simulink library "Defined_Functionality"  (R2018a)
settings: Solver=ode45  StartTime=0.0  StopTime=10.0  RelTol=1e-3
undefined symbols (not defined in the file or in its folder): IPTc_dbgsw_pct_RestoreCellSoc, IPTc_dbgval_RestoreCellSoc, IPTc_flter_PosCtrVoltRef1_front, IPTc_Gain_BCSBattVolt, IPTc_Gain_CC2, IPTc_Gain_CMLChagrMaxOptCur, IPTc_Gain_PCBTemp, IPTc_Offset_BCSBattVolt, IPTc_Offset_CC2, IPTc_Offset_CMLChagrMaxOptCur, IPTc_Offset_PCBTemp, IPTc_tm_VehShutBCUCmdDeb, IPTc_v_ChaWake_HysisDnLimit, IPTc_v_ChaWake_HysisUpLimit
settings Model: Creator=Administrator  LastModifiedBy=dhw059
settings DataIOCC: LimitDataPoints=on  SaveFormat=Array  SignalLoggingSaveFormat=ModelDataLogs
settings OptimizationCC: BlockReduction=off  BooleanDataType=off  ExpressionDepthLimit=2147483647  LifeSpan=inf
settings DebuggingCC: SaveWithParameterizedLinksMsg=none  UnderspecifiedInitializationDetection=Classic  MergeDetectMultiDrivingBlocksExec=none  SignalResolutionControl=TryResolveAllWithWarning  FcnCallInpInsideContextMsg=warning  StateNameClashWarn=warning  SFUnexpectedBacktrackingDiag=warning  SFNoUnconditionalDefaultTransitionDiag=warning  SFExecutionAtInitializationDiag=none
settings HardwareCC: ProdBitPerPointer=32  ProdBitPerSizeT=32  ProdBitPerPtrDiffT=32  ProdLargestAtomicFloat=None  ProdIntDivRoundTo=Undefined  ProdEndianess=Unspecified  ProdWordSize=32  ProdHWDeviceType=32-bit Generic  TargetUnknown=on
settings ModelReferenceCC: PropagateSignalLabelsOutOfModel=off
settings CodeAppCC: StateflowObjectComments=on
settings GRTTargetCC: TargetLangStandard=C89/C90 (ANSI)  GeneratePreprocessorConditionals=Disable all  CombineOutputUpdateFcns=off  GRTInterface=on
settings ConfigComp: CovMetricSettings=dw  CovHtmlReporting=on  CovSaveCumulativeToWorkspaceVar=on  CovSaveSingleToWorkspaceVar=on  CovExternalEMLEnable=off

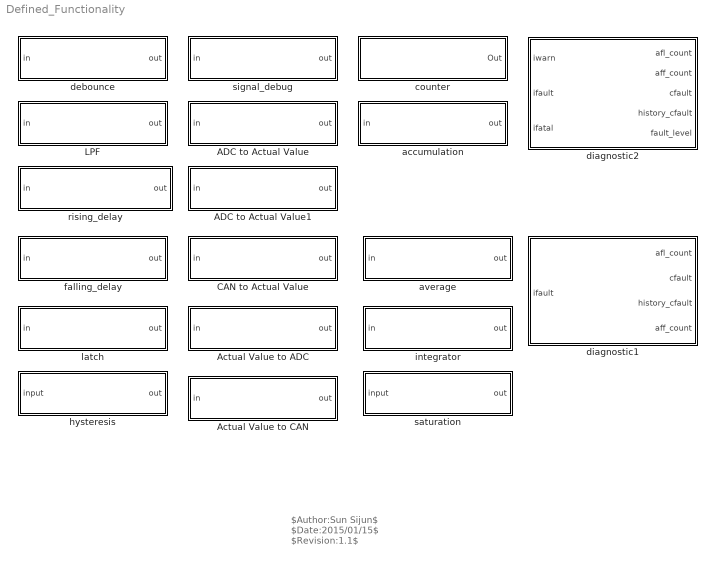
== system Defined_Functionality ==
  note: $Author:Sun Sijun$
      | $Date:2015/01/15$
      | $Revision:1.1$
  ADC to Actual Value : Subsystem  TreatAsAtomicUnit=on  RTWFcnName=ADC_CONVERSION_A_ACT  mask(Value Conversion){gain=IPTc_Gain_CC2, offset=IPTc_Offset_CC2}
      mask help:
      | To convert ADC vaule into actual value.
      | ACT=ADC*GAIN+OFFSET
      settings: AttributesFormatString=[GAIN=%<gain>]\n[OFFSET=%<offset>]  RTWFcnNameOpts=User specified
      mask Display:
      | color('black');
      | disp('CONVERSION_A');
      | port_label('input',1,'ADC')
      | port_label('output',1,'ACT')
  ADC to Actual Value1 : Subsystem  TreatAsAtomicUnit=on  RTWFcnName=ADC_CONVERSION_B_ACT21  mask(Value Conversion){offset=IPTc_Offset_PCBTemp, gain=IPTc_Gain_PCBTemp}
      mask help:
      | To convert ADC vaule into actual value.
      | ACT=(ADC+OFFSET)*GAIN
      settings: AttributesFormatString=[OFFSET=%<offset>]\n[GAIN=%<gain>]  RTWFcnNameOpts=User specified
      mask Display:
      | color('black');
      | disp('CONVERSION_B');
      | port_label('input',1,'ADC')
      | port_label('output',1,'ACT')
  Actual Value to ADC : Subsystem  TreatAsAtomicUnit=on  RTWFcnName=ACT_CONVERSION_ADC  mask(Value Conversion){gain=0, offset=0}
      mask help:
      | To convert actual value into ADC value.
      | ADC=(ACT-OFFSET)/GAIN
      settings: AttributesFormatString=[GAIN=%<gain>]\n[OFFSET=%<offset>]  RTWFcnNameOpts=User specified
      mask Display:
      | color('black');
      | disp('CONVERSION');
      | port_label('input',1,'ACT')
      | port_label('output',1,'ADC')
  Actual Value to CAN : Subsystem  TreatAsAtomicUnit=on  RTWFcnName=ACT_CONVERSION_CAN  mask(Value Conversion){gain=IPTc_Gain_BCSBattVolt, offset=IPTc_Offset_BCSBattVolt}
      mask help: To convert actual value into CAN signal.
      settings: AttributesFormatString=[GAIN=%<gain>]\n[OFFSET=%<offset>]  RTWFcnNameOpts=User specified
      mask Display:
      | color('black');
      | disp('CONVERSION');
      | port_label('input',1,'ACT')
      | port_label('output',1,'CAN')
  CAN to Actual Value : Subsystem  TreatAsAtomicUnit=on  RTWFcnName=CAN_CONVERSION_ACT  mask(Value Conversion){gain=IPTc_Gain_CMLChagrMaxOptCur, offset=IPTc_Offset_CMLChagrMaxOptCur}
      mask help:
      | To convert CAN signal into actual value.
      | ACT=CAN*GAIN+OFFSET.
      settings: AttributesFormatString=[GAIN=%<gain>]\n[OFFSET=%<offset>]  RTWFcnNameOpts=User specified
      mask Display:
      | color('black');
      | disp('CONVERSION');
      | port_label('input',1,'CAN')
      | port_label('output',1,'ACT')
  LPF : Subsystem  TreatAsAtomicUnit=on  RTWFcnName=low_pass_filter2  mask(LPF){filter_gain=IPTc_flter_PosCtrVoltRef1_front}
      mask prompts: filter_gain "LPF_GAIN"
      mask help: Low pass filter.The LPF_GAIN is positive but less than 1.
      settings: AttributesFormatString=[FILTER_GAIN=%<filter_gain>]  RTWFcnNameOpts=User specified
      mask Display:
      | disp('LPF')
      | port_label('input',1,'in')
      | port_label('output',1,'out')
  accumulation : Subsystem  TreatAsAtomicUnit=on  RTWFcnName=accumulation  mask(accumulation){Num_Threshold_Up=200, Num_Threshold_Down=0, Inc=1, Dec=0}
      mask prompts: Num_Threshold_Up "Threshold_Up"; Num_Threshold_Down "Threshold_Down"; Inc "Increment"; Dec "Decrement"
      mask help:
      | The initial output of the block is FALSE.When the input value is TRUE,the counter would increase
      | by Increment value per period,the block will not output TURE until the counter is not less than
      | Threshold.When the input value become FALSE,the counter would decrease by decrement value per
      | period,the block will not output FASLE until the counter is not more than zero.
      settings: AttributesFormatString=[THRESHOLD_UP=%<Num_Threshold_Up>]\n[THRESHOLD_DOWN=%<Num_Threshold_Down>]\n[INCREMENT=%<Inc>]\n[DECREMENT=%<Dec>]  RTWFcnNameOpts=User specified
      mask Display:
      | disp('ACCUMULATION')
      | port_label('input',1,'in')
      | port_label('output',1,'out')
  average : Subsystem  TreatAsAtomicUnit=on  RTWFcnName=average2  mask(average){time=uint16(2000), period=uint16(10)}
      mask prompts: time "Time_ms"; period "Period_ms"
      mask help: To get the average avlue of input signal in the period Time_ms.
      settings: AttributesFormatString=[TIME_ms=%<time>]\n[PERIOD_ms=%<period>]  RTWFcnNameOpts=User specified
      mask Display:
      | port_label('input',1,'in')
      | port_label('output',1,'out')
      | disp('AVERAGE')
  counter : Subsystem  TreatAsAtomicUnit=on  RTWFcnName=counter  mask(counter){initial_value=1, counter_limit=10}
      mask prompts: initial_value "Initial_Counter_Value"
      mask help: The block is a counter.It counts from initial counter value until counter limit,then it will count from initial counter value.
      settings: AttributesFormatString=[INITIAL_VALUE=%<initial_value>]\n[COUNTER_LIMIT=%<counter_limit>]  RTWFcnNameOpts=User specified
      mask Display:
      | disp('COUNTER')
      | port_label('output',1,'out')
  debounce : Subsystem  TreatAsAtomicUnit=on  RTWFcnName=debounce  mask(debounce){debounce_time=IPTc_tm_VehShutBCUCmdDeb}
      mask prompts: debounce_time "debounce_time_ms"
      mask help: Debounce the input digital signal.
      settings: AttributesFormatString=[DEBOUNCE_TIME=%<debounce_time>]  RTWFcnNameOpts=User specified
      mask Display:
      | disp('DEBOUNCE')
      | port_label('input',1,'in')
      | port_label('output',1,'out')
  diagnostic1 : Subsystem  TreatAsAtomicUnit=on  RTWFcnName=diagnostic  mask(Fault_Diagnostic){afl_inc=3, afl_dec=3, afl_threshold=10, aff_threshold=255}
      mask prompts: afl_inc "AFL_INCREMENT"; afl_dec "AFL_DECREMENT"
      mask help:
      | AFL:Accumulated Failure Level.
      | AFF:Accumulated Failure Frequency
      | AFL_INCREMENT:The value of the internal counter gets incremented each cycle if the ifault is active [uint8] [0...255].
      | AFL_DECREMENT:The value of  the internal counter gets decremented each cycle if the ifault is inactive [uint8] [0...255].
      | AFL_THRESHOLD:When the internal counter is more than AFL_THRESHOLD,fault is confirmed.
      | AFF_THRESHOLD:The aff_count must be less than AFF_THRESHOLD.
      settings: AttributesFormatString=[AFL_INCREMENT=%<afl_inc>]\n[AFL_DECREMENT=%<afl_dec>]\n[AFL_THRESHOLD=%<afl_threshold>]\n[AFF_THRESHOLD=%<aff_threshold>]  RTWFcnNameOpts=User specified
      mask Display:
      | disp('DIAGNOSTIC')
      | port_label('input',1,'ifault')
      | port_label('output',1,'afl_count')
      | port_label('output',2,'cfault')
      | port_label('output',3,'history_cfault')
      | port_label('output',4,'aff_count')
  diagnostic2 : Subsystem  TreatAsAtomicUnit=on  RTWFcnName=diagnostic  mask(Fault_Diagnostic){afl_inc=3, afl_dec=3, afl_threshold=10, aff_threshold=255}
      mask prompts: afl_inc "AFL_INCREMENT"; afl_dec "AFL_DECREMENT"
      mask help:
      | AFL:Accumulated Failure Level.
      | AFF:Accumulated Failure Frequency
      | AFL_INCREMENT:The value of the internal counter gets incremented each cycle if the ifault is active [uint8] [0...255].
      | AFL_DECREMENT:The value of  the internal counter gets decremented each cycle if the ifault is inactive [uint8] [0...255].
      | AFL_THRESHOLD:When the internal counter is more than AFL_THRESHOLD,fault is confirmed.
      | AFF_THRESHOLD:The aff_count must be less than AFF_THRESHOLD.
      settings: AttributesFormatString=[AFL_INCREMENT=%<afl_inc>]\n[AFL_DECREMENT=%<afl_dec>]\n[AFL_THRESHOLD=%<afl_threshold>]\n[AFF_THRESHOLD=%<aff_threshold>]  RTWFcnNameOpts=User specified
      mask Display:
      | disp('DIAGNOSTIC')
      | port_label('input',1,'iwarn')
      | port_label('input',2,'ifault')
      | port_label('input',3,'ifatal')
      | port_label('output',1,'afl_count')
      | port_label('output',2,'aff_count')
      | port_label('output',3,'cfault')
      | port_label('output',4,'history_cfault')
      | port_label('output',5,'fault_level')
  falling_delay : Subsystem  TreatAsAtomicUnit=on  RTWFcnName=falling_edge_delay  mask(falling edge delay){delay_time=50}
      mask prompts: delay_time "delay_time_ms"
      mask help: When the input equals TRUE,output TURE,but if the input equals FALSE,The output is delayed for delay_time_ms.
      settings: AttributesFormatString=[DELAY_TIME=%<delay_time>]  RTWFcnNameOpts=User specified
      mask Display:
      | disp('FALL_DEGE_DELAY')
      | port_label('input',1,'in')
      | port_label('output',1,'out')
  hysteresis : Subsystem  TreatAsAtomicUnit=on  RTWFcnName=hysteresis  mask(hysterisis){upper_limit=IPTc_v_ChaWake_HysisUpLimit, lower_limit=IPTc_v_ChaWake_HysisDnLimit}
      mask help: Output the specified 'on' or 'off' value by comparing the input to the specified thresholds. The on/off state of the hysteresis is not affected by input between the upper and lower limits.
      settings: AttributesFormatString=[UPPER_LIMIT=%<upper_limit>]\n[LOWER_LIMIT=%<lower_limit>]  RTWFcnNameOpts=User specified
      mask Display:
      | port_label('input',1,'in')
      | port_label('output',1,'out')
      | disp('HYSTERESIS')
  integrator : Subsystem  TreatAsAtomicUnit=on  RTWFcnName=Integrator  mask(Integrator){Initial_Value=0}
      mask prompts: Initial_Value "Initial Value of Unit Delay"
      mask help: Integrator
      settings: RTWFcnNameOpts=User specified
      mask Display:
      | disp('INTEGRATOR')
      | port_label('input',1,'in')
      | port_label('output',1,'out')
  latch : Subsystem  TreatAsAtomicUnit=on  RTWFcnName=latch  mask(Latch){}
      mask help: Latch the input value.Initial output is FALSE and then latches TRUE when the input is TRUE.
      settings: RTWFcnNameOpts=User specified
      mask Display:
      | disp('LATCH')
      | port_label('input',1,'in')
      | port_label('output',1,'out')
  rising_delay : Subsystem  TreatAsAtomicUnit=on  RTWFcnName=rising_edge_delay  mask(rising edge delay){delay_time=100}
      mask prompts: delay_time "delay_time_ms"
      mask help: When the input equals FALSE,output FALSE,but if the input equals TRUE,The output is delayed for delay_time_ms.
      settings: AttributesFormatString=[DELAY_TIME=%<delay_time>]  RTWFcnNameOpts=User specified
      mask Display:
      | disp('RISING_DEGE_DELAY')
      | port_label('input',1,'in')
      | port_label('output',1,'out')
  saturation : Subsystem  TreatAsAtomicUnit=on  RTWFcnName=saturation  mask(saturation){upper_limit=2, lower_limit=0}
      mask help: Limit input signal to the upper and lower saturation values.
      settings: AttributesFormatString=[UPPER_LIMIT=%<upper_limit>]\n[LOWER_LIMIT=%<lower_limit>]  RTWFcnNameOpts=User specified
      mask Display:
      | port_label('input',1,'in')
      | port_label('output',1,'out')
      | disp('SATURATION')
  signal_debug : Subsystem  TreatAsAtomicUnit=on  RTWFcnName=Signal_Debug  mask(signal debug){debug_switch=IPTc_dbgsw_pct_RestoreCellSoc, debug_value=IPTc_dbgval_RestoreCellSoc}
      mask help: To debug signal.
      settings: AttributesFormatString=[SWITCH=%<debug_switch>]\n[VALUE=%<debug_value>]  RTWFcnNameOpts=User specified
      mask Display:
      | port_label('input',1,'in')
      | port_label('output',1,'out')
      | disp('SIGNAL_DEBUG')

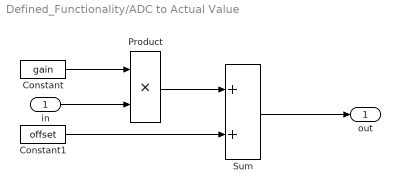
== system Defined_Functionality/ADC to Actual Value ==
  in : Inport
  Constant : Constant  Value=gain
  Constant1 : Constant  Value=offset
  Product : Product  OutDataTypeStr=fixdt(1,16,4)  RndMeth=Zero
  Sum : Sum  OutDataTypeStr=fixdt(1,16,4)
  out : Outport
  wires:
  Constant/1 -> Product/1
  in/1 -> Product/2
  Product/1 -> Sum/1
  Sum/1 -> out/1
  Constant1/1 -> Sum/2

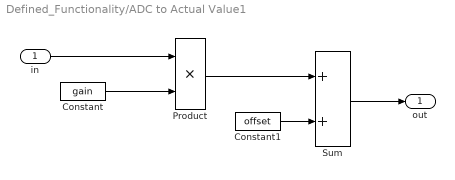
== system Defined_Functionality/ADC to Actual Value1 ==
  in : Inport
  Constant : Constant  Value=gain
  Constant1 : Constant  Value=offset
  Product : Product  OutDataTypeStr=fixdt(1,16,4)  RndMeth=Zero
  Sum : Sum  OutDataTypeStr=int16
  out : Outport
  wires:
  in/1 -> Product/1
  Product/1 -> Sum/1
  Sum/1 -> out/1
  Constant1/1 -> Sum/2
  Constant/1 -> Product/2

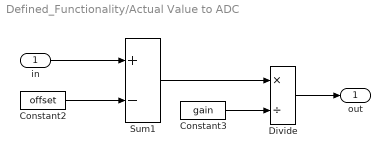
== system Defined_Functionality/Actual Value to ADC ==
  in : Inport
  Constant2 : Constant  Value=offset
  Constant3 : Constant  Value=gain  OutDataTypeStr=fixdt(1,32,0.0001,0)
  Divide : Product  Inputs=*/  OutDataTypeStr=uint16  RndMeth=Zero
  Sum1 : Sum  Inputs=+-  OutDataTypeStr=fixdt(1,32,0.0001,0)
  out : Outport
  wires:
  Divide/1 -> out/1
  Constant3/1 -> Divide/2
  Sum1/1 -> Divide/1
  Constant2/1 -> Sum1/2
  in/1 -> Sum1/1

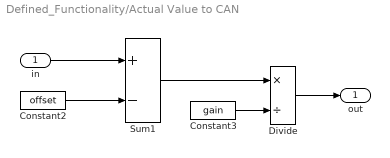
== system Defined_Functionality/Actual Value to CAN ==
  in : Inport
  Constant2 : Constant  Value=offset
  Constant3 : Constant  Value=gain
  Divide : Product  Inputs=*/  OutDataTypeStr=Inherit: Inherit via back propagation  RndMeth=Zero
  Sum1 : Sum  Inputs=+-
  out : Outport
  wires:
  in/1 -> Sum1/1
  Constant2/1 -> Sum1/2
  Sum1/1 -> Divide/1
  Constant3/1 -> Divide/2
  Divide/1 -> out/1

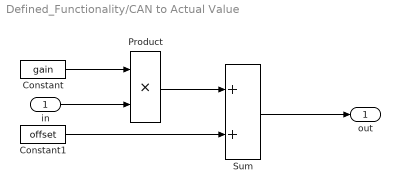
== system Defined_Functionality/CAN to Actual Value ==
  in : Inport
  Constant : Constant  Value=gain
  Constant1 : Constant  Value=offset
  Product : Product  OutDataTypeStr=fixdt(1,16,4)  RndMeth=Zero
  Sum : Sum  OutDataTypeStr=fixdt(1,16,4)
  out : Outport
  wires:
  Constant1/1 -> Sum/2
  Sum/1 -> out/1
  Product/1 -> Sum/1
  in/1 -> Product/2
  Constant/1 -> Product/1

== system Defined_Functionality/LPF ==
  in : Inport
  Low_Pass_Filter : Subsystem
  Unit Delay : UnitDelay  SampleTime=-1
  out : Outport
  wires:
  in/1 -> Low_Pass_Filter/2(input)
  Unit Delay/1 -> Low_Pass_Filter/1(pre_output)
  Low_Pass_Filter/1(output) -> Unit Delay/1, out/1

== system Defined_Functionality/accumulation ==
  in : Inport
  accumulation : Stateflow chart  TreatAsAtomicUnit=on
  out : Outport
  wires:
  accumulation/1(out) -> out/1
  in/1 -> accumulation/1(in)

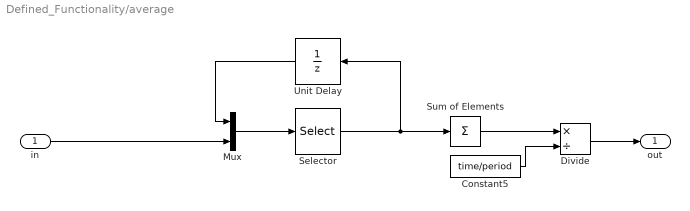
== system Defined_Functionality/average ==
  in : Inport
  Constant5 : Constant  Value=time/period
  Divide : Product  Inputs=*/  OutDataTypeStr=fixdt(1,16,5)
  Mux : Mux  Inputs=2
  Selector : Selector  InputPortWidth=time/period+1  IndexOptions=Index vector (dialog)  Indices=[2:time/period+1]  OutputSizes=1
  Sum of Elements : Sum  Inputs=+  OutDataTypeStr=fixdt(1,32,6)
  Unit Delay : UnitDelay  SampleTime=-1
  out : Outport
  wires:
  Unit Delay/1 -> Mux/1
  Selector/1 -> Sum of Elements/1, Unit Delay/1
  in/1 -> Mux/2
  Mux/1 -> Selector/1
  Divide/1 -> out/1
  Sum of Elements/1 -> Divide/1
  Constant5/1 -> Divide/2

== system Defined_Functionality/counter ==
  counter : Stateflow chart  TreatAsAtomicUnit=on
  Out : Outport
  wires:
  counter/1(out) -> Out/1

== system Defined_Functionality/debounce ==
  in : Inport
  debounce : Stateflow chart  TreatAsAtomicUnit=on
  out : Outport
  wires:
  debounce/1(out) -> out/1
  in/1 -> debounce/1(in)

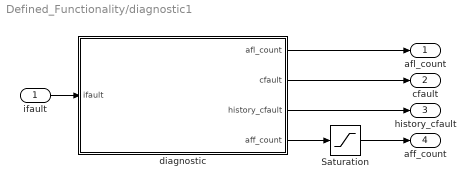
== system Defined_Functionality/diagnostic1 ==
  ifault : Inport
  Saturation : Saturate  UpperLimit=aff_threshold  LowerLimit=0
  diagnostic : Stateflow chart  TreatAsAtomicUnit=on
  afl_count : Outport
  cfault : Outport  Port=2
  history_cfault : Outport  Port=3
  aff_count : Outport  Port=4
  wires:
  ifault/1 -> diagnostic/1(ifault)
  diagnostic/1(afl_count) -> afl_count/1
  diagnostic/2(cfault) -> cfault/1
  diagnostic/3(history_cfault) -> history_cfault/1
  diagnostic/4(aff_count) -> Saturation/1
  Saturation/1 -> aff_count/1

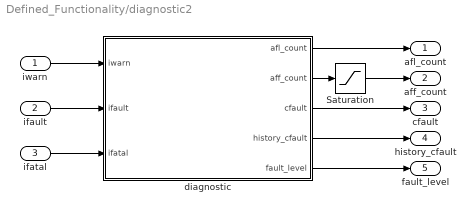
== system Defined_Functionality/diagnostic2 ==
  iwarn : Inport
  ifault : Inport  Port=2
  ifatal : Inport  Port=3
  Saturation : Saturate  UpperLimit=aff_threshold  LowerLimit=0
  diagnostic : Stateflow chart  TreatAsAtomicUnit=on
  afl_count : Outport
  aff_count : Outport  Port=2
  cfault : Outport  Port=3
  history_cfault : Outport  Port=4
  fault_level : Outport  Port=5
  wires:
  diagnostic/5(fault_level) -> fault_level/1
  ifatal/1 -> diagnostic/3(ifatal)
  iwarn/1 -> diagnostic/1(iwarn)
  ifault/1 -> diagnostic/2(ifault)
  diagnostic/1(afl_count) -> afl_count/1
  diagnostic/3(cfault) -> cfault/1
  diagnostic/4(history_cfault) -> history_cfault/1
  diagnostic/2(aff_count) -> Saturation/1
  Saturation/1 -> aff_count/1

== system Defined_Functionality/falling_delay ==
  in : Inport
  edge_delay : Stateflow chart  TreatAsAtomicUnit=on
  out : Outport
  wires:
  edge_delay/1(out) -> out/1
  in/1 -> edge_delay/1(in)

== system Defined_Functionality/hysteresis ==
  input : Inport
  Data Type Conversion : DataTypeConversion  OutDataTypeStr=boolean
  Relay : Relay  OnSwitchValue=upper_limit  OffSwitchValue=lower_limit  OutDataTypeStr=int8
  out : Outport
  wires:
  input/1 -> Relay/1
  Relay/1 -> Data Type Conversion/1
  Data Type Conversion/1 -> out/1

== system Defined_Functionality/integrator ==
  in : Inport
  Add4 : Sum
  Unit Delay1 : UnitDelay  InitialCondition=Initial_Value  SampleTime=-1
  out : Outport
  wires:
  in/1 -> Add4/2
  Add4/1 -> Unit Delay1/1, out/1
  Unit Delay1/1 -> Add4/1

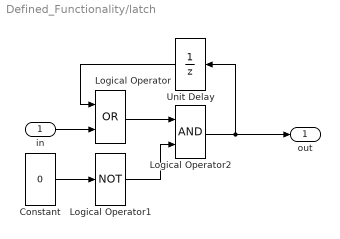
== system Defined_Functionality/latch ==
  in : Inport
  Constant : Constant  Value=0  OutDataTypeStr=boolean
  Logical Operator : Logic  Operator=OR  AllPortsSameDT=off  OutDataTypeStr=boolean
  Logical Operator1 : Logic  Operator=NOT  AllPortsSameDT=off  OutDataTypeStr=boolean
  Logical Operator2 : Logic  AllPortsSameDT=off  OutDataTypeStr=boolean
  Unit Delay : UnitDelay  SampleTime=-1
  out : Outport
  wires:
  Logical Operator2/1 -> Unit Delay/1, out/1
  Unit Delay/1 -> Logical Operator/1
  Logical Operator1/1 -> Logical Operator2/2
  Logical Operator/1 -> Logical Operator2/1
  Constant/1 -> Logical Operator1/1
  in/1 -> Logical Operator/2

== system Defined_Functionality/rising_delay ==
  in : Inport
  edge_delay : Stateflow chart  TreatAsAtomicUnit=on
  out : Outport
  wires:
  in/1 -> edge_delay/1(in)
  edge_delay/1(out) -> out/1

== system Defined_Functionality/saturation ==
  input : Inport
  Saturation : Saturate  UpperLimit=upper_limit  LowerLimit=lower_limit
  out : Outport
  wires:
  input/1 -> Saturation/1
  Saturation/1 -> out/1

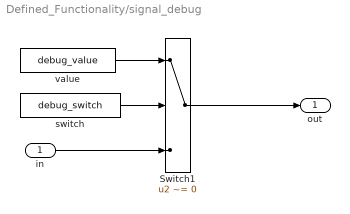
== system Defined_Functionality/signal_debug ==
  in : Inport
  Switch1 : Switch  Criteria=u2 ~= 0  Threshold=0.5
  switch : Constant  Value=debug_switch  OutDataTypeStr=boolean
  value : Constant  Value=debug_value
  out : Outport
  wires:
  value/1 -> Switch1/1
  in/1 -> Switch1/3
  Switch1/1 -> out/1
  switch/1 -> Switch1/2

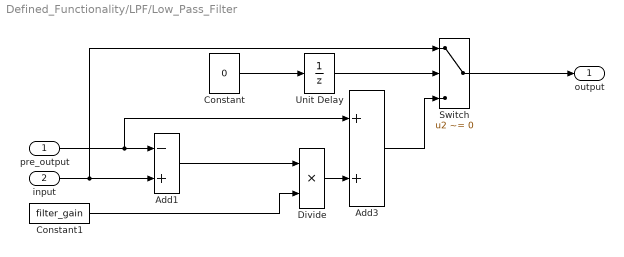
== system Defined_Functionality/LPF/Low_Pass_Filter ==
  pre_output : Inport
  input : Inport  Port=2
  Add1 : Sum  Inputs=-+  OutDataTypeStr=fixdt(1,16,4)
  Add3 : Sum  OutDataTypeStr=fixdt(1,16,4)
  Constant : Constant  Value=0  OutDataTypeStr=boolean
  Constant1 : Constant  Value=filter_gain
  Divide : Product  Inputs=**  OutDataTypeStr=fixdt(1,16,4)
  Switch : Switch  Criteria=u2 ~= 0
  Unit Delay : UnitDelay  InitialCondition=1  SampleTime=-1
  output : Outport
  wires:
  Switch/1 -> output/1
  Constant/1 -> Unit Delay/1
  Unit Delay/1 -> Switch/2
  Add3/1 -> Switch/3
  Divide/1 -> Add3/2
  Add1/1 -> Divide/1
  Constant1/1 -> Divide/2
  input/1 -> Switch/1, Add1/2
  pre_output/1 -> Add3/1, Add1/1

== stateflow chart Defined_Functionality/rising_delay/edge_delay ==
  state COUNTER
    (default) -> (junction 19) : {counter=1;}
    COUNTER -> (junction 19) [order 1]
    (junction 19) -> (junction 20) : {counter+=10;}
  state INITIAL_STATE
    entry: out=0;
  state FINAL_STATE
    entry: out=1;
  (default) -> INITIAL_STATE
  INITIAL_STATE -> COUNTER : [in==1]
  COUNTER -> INITIAL_STATE [order 2] : [in==0]
  COUNTER -> FINAL_STATE [order 1] : [in!=0&&counter>=delay_time]
  FINAL_STATE -> INITIAL_STATE : [in==0]
  data: in input boolean; out output boolean; counter local uint16; delay_time parameter uint16

== stateflow chart Defined_Functionality/debounce/debounce ==
  state No_Debounce
    (default) -> (junction 99)
    (junction 99) -> (junction 100) : {out=in;}
    No_Debounce -> (junction 99) [order 1]
  state Debounce
    state Wait
      state To_on
        (default) -> (junction 77) : {Timer_On=1;}
        (junction 77) -> (junction 78) : {Timer_On++;}
        To_on -> (junction 77) [order 1]
      state To_off
        (default) -> (junction 79) : {Timer_Off=1;}
        (junction 79) -> (junction 80) : {Timer_Off++;}
        To_off -> (junction 79) [order 1]
    state FALSE
      entry: out=0;
    state TURE
      entry: out=1;
    (default) -> FALSE
    FALSE -> To_on [order 2] : [in==1]
    To_on -> (junction 81) [order 1] : [10*Timer_On>=debounce_time&&in!=0]
    (junction 81) -> TURE
    To_on -> FALSE [order 2] : [in==0]
    (junction 82) -> FALSE
    To_off -> (junction 82) [order 2] : [10*Timer_Off>=debounce_time&&in!=1]
    TURE -> To_off : [in==0]
    To_off -> TURE [order 1] : [in==1]
  (default) -> Debounce
  FALSE -> No_Debounce [order 1] : [debounce_time==0]
  No_Debounce -> FALSE [order 1] : [debounce_time!=0]
  data: in input boolean; out output boolean; count_timer local uint16; Timer_Off local uint16; Timer_On local uint16; debounce_time parameter uint16

== stateflow chart Defined_Functionality/falling_delay/edge_delay ==
  state COUNTER
    (default) -> (junction 19) : {counter=1;}
    COUNTER -> (junction 19) [order 1]
    (junction 19) -> (junction 20) : {counter+=10;}
  state INITIAL_STATE
    entry: out=1;
  state FINAL_STATE
    entry: out=0;
  (default) -> INITIAL_STATE
  INITIAL_STATE -> COUNTER : [in==0]
  COUNTER -> INITIAL_STATE [order 2] : [in==1]
  COUNTER -> FINAL_STATE [order 1] : [in!=1&&counter>=delay_time]
  FINAL_STATE -> INITIAL_STATE : [in==1]
  data: in input boolean; out output boolean; counter local uint16; delay_time parameter uint16

== stateflow chart Defined_Functionality/counter/counter ==
  state COUNTER
    (default) -> (junction 19) : {counter=initial_value;}
    COUNTER -> (junction 19) [order 1]
    (junction 19) -> (junction 20) : {out=counter;counter+=1;}
  (default) -> COUNTER
  (junction 54) -> COUNTER
  COUNTER -> (junction 49) [order 1] : [out>=counter_limit]
  (junction 49) -> (junction 54)
  data: out output uint16; counter local uint16; initial_value parameter uint16; counter_limit parameter uint16

== stateflow chart Defined_Functionality/diagnostic2/diagnostic ==
  state Fault_Diagnostic
    state Counter
      state AFL_INC
        (default) -> (junction 19)
        (junction 19) -> (junction 20) : {afl_count=counter;counter+=afl_inc;}
        AFL_INC -> (junction 19) [order 1]
      state AFL_DEC
        (default) -> (junction 21)
        (junction 21) -> (junction 22) : {afl_count=counter;counter-=afl_dec;}
        AFL_DEC -> (junction 21) [order 1]
      AFL_INC -> AFL_DEC [order 2] : [iwarn==0&&...
          | ifault==0&&...
          | ifatal==0&&...
          | counter<afl_threshold]
      AFL_DEC -> AFL_INC [order 2] : [(iwarn==1||...
          | ifault==1||...
          | ifatal==1)&&...
          | counter>0]
    state No_Cfault
      entry: cfault=0;
      counter=0;
      fault_level=0;
      afl_count=counter;
    state Cfault
      (default) -> (junction 164) : {afl_count=afl_threshold;
          | counter=afl_threshold;
          | cfault=1;
          | history_cfault=1;
          | aff_count++;}
      (junction 164) -> (junction 166) [order 1] : [iwarn==1]
      (junction 166) -> (junction 170) : {fault_level = 1;}
      (junction 164) -> (junction 170) [order 2]
      (junction 170) -> (junction 168) [order 1] : [ifault==1]
      (junction 168) -> (junction 176) : {fault_level = 2;}
      (junction 170) -> (junction 176) [order 2]
      (junction 176) -> (junction 174) [order 1] : [ifatal==1]
      (junction 174) -> (junction 181) : {fault_level = 3;}
      (junction 176) -> (junction 181) [order 2]
      (junction 181) -> (junction 179)
    (default) -> No_Cfault : {aff_count=0;}
    No_Cfault -> AFL_INC : [iwarn==1||...
        | ifault==1||...
        | ifatal==1]
    AFL_INC -> (junction 104) [order 1] : [counter>=afl_threshold]
    (junction 104) -> Cfault
    (junction 102) -> No_Cfault
    AFL_DEC -> (junction 102) [order 1] : [counter<=0]
    Cfault -> AFL_DEC : [iwarn==0&&...
        | ifault==0&&...
        | ifatal==0]
  (default) -> Fault_Diagnostic
  data: iwarn input boolean; afl_count output int16; aff_count output uint8; afl_dec parameter uint8; afl_inc parameter uint8; afl_threshold parameter uint8; cfault output boolean; history_cfault output boolean; ifault input boolean; aff_threshold parameter uint8; counter local int16; ifatal input boolean; fault_level output uint8

== stateflow chart Defined_Functionality/diagnostic1/diagnostic ==
  state Fault_Diagnostic
    state Counter
      state AFL_INC
        (default) -> (junction 19)
        (junction 19) -> (junction 20) : {afl_count=counter;counter+=afl_inc;}
        AFL_INC -> (junction 19) [order 1]
      state AFL_DEC
        (default) -> (junction 21)
        (junction 21) -> (junction 22) : {afl_count=counter;counter-=afl_dec;}
        AFL_DEC -> (junction 21) [order 1]
      AFL_INC -> AFL_DEC [order 2] : [ifault==0&&...
          | counter<afl_threshold]
      AFL_DEC -> AFL_INC [order 2] : [ifault==1&&...
          | counter>0]
    state No_Cfault
      entry: cfault=0;
      counter=0;
      afl_count=counter;
    state Cfault
      entry: afl_count=afl_threshold;
      counter=afl_threshold;
      cfault=1;
      history_cfault=1;
      aff_count++;
    (default) -> No_Cfault : {aff_count=0;}
    No_Cfault -> AFL_INC : [ifault==1]
    AFL_INC -> (junction 104) [order 1] : [counter>=afl_threshold]
    (junction 104) -> Cfault
    (junction 102) -> No_Cfault
    AFL_DEC -> (junction 102) [order 1] : [counter<=0]
    Cfault -> AFL_DEC : [ifault==0]
  state No_Fault_Diagnostic
    (default) -> (junction 89)
    (junction 89) -> (junction 90) : {cfault = 0;
        | afl_count = 0;
        | history_cfault = 0;
        | aff_count = 0;}
    No_Fault_Diagnostic -> (junction 89) [order 1]
  (default) -> No_Fault_Diagnostic
  No_Fault_Diagnostic -> Fault_Diagnostic [order 1] : [afl_threshold!=0]
  Fault_Diagnostic -> No_Fault_Diagnostic : [afl_threshold==0]
  data: afl_count output int16; afl_dec parameter uint8; afl_inc parameter uint8; afl_threshold parameter uint8; cfault output boolean; history_cfault output boolean; ifault input boolean; aff_count output uint8; counter local int16

== stateflow chart Defined_Functionality/accumulation/accumulation ==
  state Accumulation
    state Counter
      state Inc
        (default) -> (junction 70)
        (junction 70) -> (junction 71) : {Num=Num+Inc;}
        Inc -> (junction 70) [order 1]
      state Dec
        (default) -> (junction 76)
        (junction 76) -> (junction 77) : {Num=Num-Dec;}
        Dec -> (junction 76) [order 1]
      Dec -> Inc [order 2] : [in==1&&...
          | Num>Num_Threshold_Down]
      Inc -> Dec [order 2] : [in==0&&...
          | Num<Num_Threshold_Up]
    state Off
      entry: out=0;
      Num=0;
    state On
      entry: out=1;
    (default) -> Off
    Off -> Inc : [in==1]
    Inc -> (junction 57) [order 1] : [Num>=Num_Threshold_Up]
    (junction 57) -> On
    (junction 58) -> Off
    On -> Dec : [in==0]
    Dec -> (junction 58) [order 1] : [Num<=Num_Threshold_Down]
  state No_Accumulation
    (default) -> (junction 84)
    (junction 84) -> (junction 85) : {out = 0;}
    No_Accumulation -> (junction 84) [order 1]
  (default) -> No_Accumulation
  No_Accumulation -> Accumulation [order 1] : [Num_Threshold_Up!=0]
  Accumulation -> No_Accumulation : [Num_Threshold_Up==0]
  data: in input boolean; out output boolean; Dec parameter uint8; Inc parameter uint8; Num local int16; Num_Threshold_Down parameter uint16; Num_Threshold_Up parameter uint16
